simulink model "punkt1"  (R2015b)
settings: Solver=VariableStepAuto  StartTime=0.0  StopTime=8  MaxStep=0.001  MinStep=0.0001  RelTol=1e-3
settings Model: Creator=hohotulca  LastModifiedBy=hohotulca

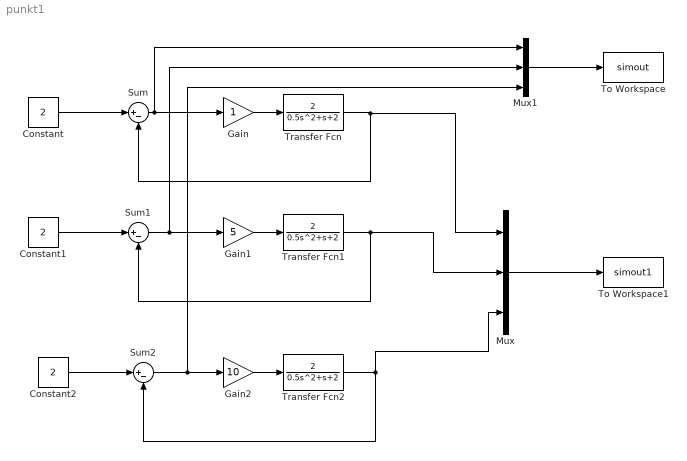
== system punkt1 ==
  Constant : Constant  Value=2
  Constant1 : Constant  Value=2
  Constant2 : Constant  Value=2
  Gain : Gain
  Gain1 : Gain  Gain=5
  Gain2 : Gain  Gain=10
  Mux : Mux  Inputs=3
  Mux1 : Mux  Inputs=3
  Sum : Sum  Inputs=|+-
  Sum1 : Sum  Inputs=|+-
  Sum2 : Sum  Inputs=|+-
  To Workspace : ToWorkspace  VariableName=simout  SaveFormat=Timeseries  SampleTime=-1
  To Workspace1 : ToWorkspace  VariableName=simout1  SaveFormat=Timeseries  SampleTime=-1
  Transfer Fcn : TransferFcn  Numerator=[2]  Denominator=[0.5 1 2]
  Transfer Fcn1 : TransferFcn  Numerator=[2]  Denominator=[0.5 1 2]
  Transfer Fcn2 : TransferFcn  Numerator=[2]  Denominator=[0.5 1 2]
  wires:
  Gain/1 -> Transfer Fcn/1
  Transfer Fcn/1 -> Mux/1, Sum/2
  Constant/1 -> Sum/1
  Gain1/1 -> Transfer Fcn1/1
  Transfer Fcn1/1 -> Sum1/2, Mux/2
  Constant1/1 -> Sum1/1
  Sum1/1 -> Mux1/2, Gain1/1
  Gain2/1 -> Transfer Fcn2/1
  Transfer Fcn2/1 -> Mux/3, Sum2/2
  Constant2/1 -> Sum2/1
  Sum2/1 -> Gain2/1, Mux1/3
  Mux/1 -> To Workspace1/1
  Sum/1 -> Gain/1, Mux1/1
  Mux1/1 -> To Workspace/1
